simulink model "LFSRinlantuitTEMA"  (R2019a)
settings: Solver=VariableStepAuto  StartTime=0.0  StopTime=10.0  RelTol=1e-3
settings Model: Creator=Maftei Silviu  LastModifiedBy=Maftei Silviu

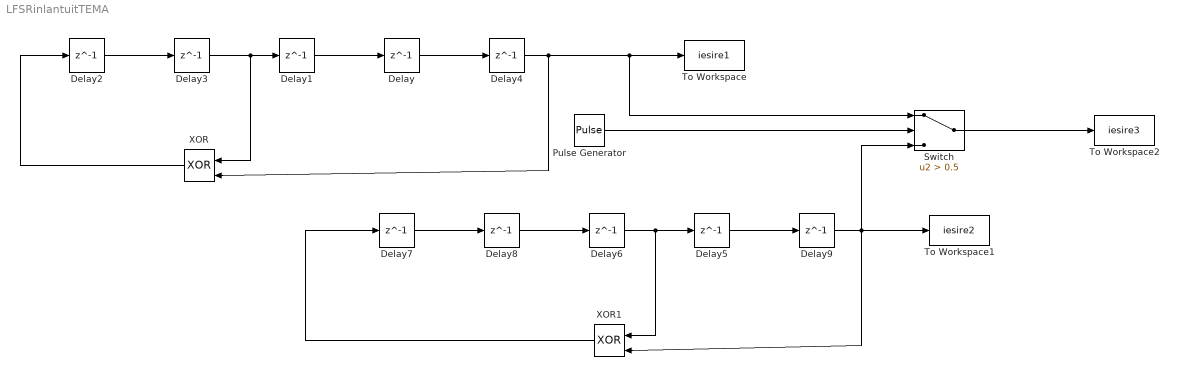
== system LFSRinlantuitTEMA ==
  Delay : Delay  DelayLength=1  InitialCondition=0
  Delay{1..4,6..9} (8 alike) : Delay  DelayLength=1  InitialCondition=1
  Delay5 : Delay  DelayLength=1  InitialCondition=0
  Pulse Generator : DiscretePulseGenerator  SampleTime=0.005
  Switch : Switch  Criteria=u2 > Threshold  Threshold=0.5
  To Workspace : ToWorkspace  VariableName=iesire1  SampleTime=0.005
      settings: Save2DSignal=2-D array (concatenate along first dimension)
  To Workspace1 : ToWorkspace  VariableName=iesire2  SampleTime=0.005
      settings: Save2DSignal=2-D array (concatenate along first dimension)
  To Workspace2 : ToWorkspace  VariableName=iesire3  SampleTime=0.005
      settings: Save2DSignal=2-D array (concatenate along first dimension)
  XOR : Logic  Operator=XOR  IconShape=distinctive  AllPortsSameDT=off  OutDataTypeStr=boolean
  XOR1 : Logic  Operator=XOR  IconShape=distinctive  AllPortsSameDT=off  OutDataTypeStr=boolean
  wires:
  Delay1/1 -> Delay/1
  XOR/1 -> Delay2/1
  Delay2/1 -> Delay3/1
  Delay3/1 -> Delay1/1, XOR/1
  Delay/1 -> Delay4/1
  Delay4/1 -> Switch/1, To Workspace/1, XOR/2
  Delay7/1 -> Delay8/1
  Delay9/1 -> Switch/3, To Workspace1/1, XOR1/2
  Delay5/1 -> Delay9/1
  XOR1/1 -> Delay7/1
  Delay8/1 -> Delay6/1
  Delay6/1 -> XOR1/1, Delay5/1
  Switch/1 -> To Workspace2/1
  Pulse Generator/1 -> Switch/2
